simulink model "ADRCsim"  (R2015b)
settings: Solver=ode45  StartTime=0.0  StopTime=10.0  RelTol=1e-3
settings Model: Creator=cly  LastModifiedBy=feiyang
settings DataIOCC: LimitDataPoints=off  SaveFormat=Array  SignalLoggingSaveFormat=ModelDataLogs  SignalLoggingName=sigsout
settings HardwareCC: ProdBitPerPointer=32  ProdLargestAtomicFloat=None  ProdIntDivRoundTo=Undefined  ProdEndianess=Unspecified  ProdWordSize=32  ProdHWDeviceType=32-bit Generic
settings GRTTargetCC: GeneratePreprocessorConditionals=Disable all
settings ConfigComp: CovModelRefEnable=Off

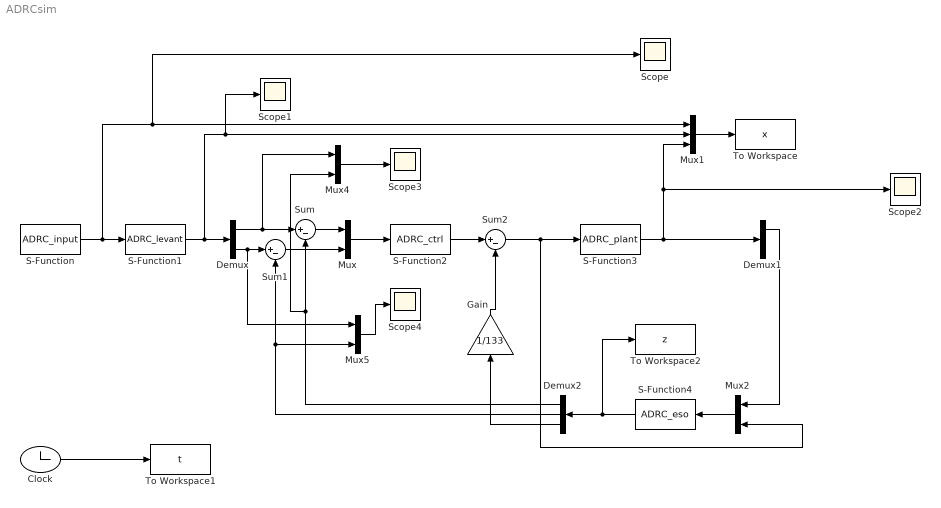
== system ADRCsim ==
  Clock : Clock
  Demux : Demux  Outputs=2
  Demux1 : Demux  Outputs=3
  Demux2 : Demux  Outputs=3
  Gain : Gain  Gain=1/133
  Mux{,2,4..5} (4 alike) : Mux  Inputs=2
  Mux1 : Mux  Inputs=3
  S-Function : S-Function  FunctionName=ADRC_input  SFunctionDeploymentMode=off  EnableBusSupport=off
  S-Function1 : S-Function  FunctionName=ADRC_levant  SFunctionDeploymentMode=off  EnableBusSupport=off
  S-Function2 : S-Function  FunctionName=ADRC_ctrl  SFunctionDeploymentMode=off  EnableBusSupport=off
  S-Function3 : S-Function  FunctionName=ADRC_plant  SFunctionDeploymentMode=off  EnableBusSupport=off
  S-Function4 : S-Function  FunctionName=ADRC_eso  SFunctionDeploymentMode=off  EnableBusSupport=off
  Scope{,1..4} (5 alike) : Scope
  Sum : Sum  Inputs=|+-
  Sum1 : Sum  Inputs=|+-
  Sum2 : Sum  Inputs=|+-
  To Workspace : ToWorkspace  VariableName=x  SampleTime=-1
  To Workspace1 : ToWorkspace  VariableName=t  SampleTime=-1
  To Workspace2 : ToWorkspace  VariableName=z  SampleTime=-1
  wires:
  S-Function/1 -> Scope/1, Mux1/1, S-Function1/1
  S-Function1/1 -> Scope1/1, Mux1/2, Demux/1
  Demux/2 -> Mux5/1, Sum1/1
  Demux/1 -> Mux4/1, Sum/1
  Sum/1 -> Mux/1
  Sum1/1 -> Mux/2
  Mux/1 -> S-Function2/1
  S-Function2/1 -> Sum2/1
  Sum2/1 -> Mux2/2, S-Function3/1
  S-Function4/1 -> To Workspace2/1, Demux2/1
  Gain/1 -> Sum2/2
  Mux2/1 -> S-Function4/1
  S-Function3/1 -> Demux1/1, Scope2/1, Mux1/3
  Mux1/1 -> To Workspace/1
  Clock/1 -> To Workspace1/1
  Demux1/1 -> Mux2/1
  Demux2/1 -> Mux4/2, Sum/2
  Demux2/2 -> Mux5/2, Sum1/2
  Demux2/3 -> Gain/1
  Mux4/1 -> Scope3/1
  Mux5/1 -> Scope4/1
